simulink subsystem "Sensoress"  (R2023b)
settings: Solver=VariableStepAuto  StartTime=0.0  StopTime=10.0  RelTol=1e-3
libraries: arduinolib x2
settings Model: Creator=marqu  LastModifiedBy=marqu

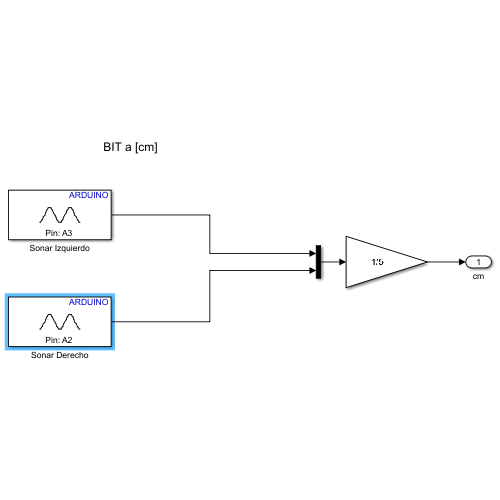
[thumbnail: Simulink's stored preview of the top-level diagram]
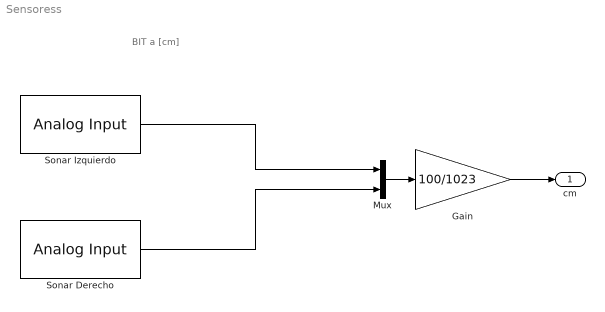
== system Sensoress ==
  note: BIT a [cm]
  Gain : Gain  Gain=100/1023
  Mux : Mux  Inputs=2
  Sonar Derecho : arduinolib/Analog Input  pinNumber=2  ReadResultsOnly=off  ConversionTriggerSource=Software  ExternalTriggerType=uint32( 0 )  OutputDataType=uint16  EnableConversionCompleteNotify=off  EnableOuputStatus=off  SampleTime=0.1  blockPlatform=arduino
  Sonar Izquierdo : arduinolib/Analog Input  pinNumber=3  ReadResultsOnly=off  ConversionTriggerSource=Software  ExternalTriggerType=uint32( 0 )  OutputDataType=uint16  EnableConversionCompleteNotify=off  EnableOuputStatus=off  SampleTime=0.1  blockPlatform=arduino
  cm : Outport
  wires:
  Gain/1 -> cm/1
  Mux/1 -> Gain/1
  Sonar Derecho/1 -> Mux/2
  Sonar Izquierdo/1 -> Mux/1
